simulink model "IEEE30_case"  (R2024b)
settings: Solver=FixedStepAuto  StartTime=0  StopTime=5  FixedStep=1e-7  RelTol=1e-3
values from neighbouring files (symbols this model uses):
  GFL_DFIG_7_C_bus = 0.08    [IEEE30_case_parameters.m]
  GFL_DFIG_7_D_mutual = 2.500000e+3    (= 2500)    [IEEE30_case_parameters.m]
  GFL_DFIG_7_f0 = 60    [IEEE30_case_parameters.m]
  GFL_DFIG_7_gPLLi = 3200    [IEEE30_case_parameters.m]
  GFL_DFIG_7_gPLLp = 650    [IEEE30_case_parameters.m]
  GFL_DFIG_7_H_WT = 0.4    [IEEE30_case_parameters.m]
  GFL_DFIG_7_Hg = 0.8    [IEEE30_case_parameters.m]
  GFL_DFIG_7_Igq_ref = 0    [IEEE30_case_parameters.m]
  GFL_DFIG_7_Ird_ref = 704.45696    [IEEE30_case_parameters.m]
  GFL_DFIG_7_KI_V = -300000    [IEEE30_case_parameters.m]
  GFL_DFIG_7_KP_V = -1000    [IEEE30_case_parameters.m]
  GFL_DFIG_7_Ksh = 1.254300e+4    (= 12543)    [IEEE30_case_parameters.m]
  GFL_DFIG_7_Lg = 0.000483    [IEEE30_case_parameters.m]
  GFL_DFIG_7_Lm_pu = 4    [IEEE30_case_parameters.m]
  GFL_DFIG_7_N = 100    [IEEE30_case_parameters.m]
  GFL_DFIG_7_p = 2    [IEEE30_case_parameters.m]
  GFL_DFIG_7_Pitch = 0    [IEEE30_case_parameters.m]
  GFL_DFIG_7_R = 44    [IEEE30_case_parameters.m]
  GFL_DFIG_7_Rg = 2.000000e-5    (= 2e-05)    [IEEE30_case_parameters.m]
  GFL_DFIG_7_rho = 1.225    [IEEE30_case_parameters.m]
  GFL_DFIG_7_rPLLi = 4500    [IEEE30_case_parameters.m]
  GFL_DFIG_7_rPLLp = 620    [IEEE30_case_parameters.m]
  GFL_DFIG_7_Rs_pu = 0.011    [IEEE30_case_parameters.m]
  GFL_DFIG_7_Sbase = 2.000000e+6    (= 2000000)    [IEEE30_case_parameters.m]
  GFL_DFIG_7_ugq_ref = 0    [IEEE30_case_parameters.m]
  GFL_DFIG_7_usd_ref = 0    [IEEE30_case_parameters.m]
  GFL_DFIG_7_Vbase = 690    [IEEE30_case_parameters.m]
  GFL_DFIG_7_Vdc_ref = 1200    [IEEE30_case_parameters.m]
  GFL_DFIG_7_wind = 12    [IEEE30_case_parameters.m]
  GFL_DFIG_7_wm_ref = 518.184209    [IEEE30_case_parameters.m]
  SG_D_13_D = 0.01056    [IEEE30_case_parameters.m]
  SG_D_13_EnableSaturation = 0    [IEEE30_case_parameters.m]
  SG_D_13_f0 = 60    [IEEE30_case_parameters.m]
  SG_D_13_H = 7.5    [IEEE30_case_parameters.m]
  SG_D_13_K_A = 20    [IEEE30_case_parameters.m]
  SG_D_13_K_E = 1.000000e+1    (= 10)    [IEEE30_case_parameters.m]
  SG_D_13_K_F = 2.363    [IEEE30_case_parameters.m]
  SG_D_13_K_s = 0.5    [IEEE30_case_parameters.m]
  SG_D_13_R_a = 0.001088    [IEEE30_case_parameters.m]
  SG_D_13_S_A = 1    [IEEE30_case_parameters.m]
  SG_D_13_S_B = 0.103    [IEEE30_case_parameters.m]
  SG_D_13_S_N = 10.659857    [IEEE30_case_parameters.m]
  SG_D_13_SpeedPara = 200    [IEEE30_case_parameters.m]
  SG_D_13_T_0 = 0.370163    [IEEE30_case_parameters.m]
  SG_D_13_T_1 = 0.3    [IEEE30_case_parameters.m]
  SG_D_13_T_2 = 0.05    [IEEE30_case_parameters.m]
  SG_D_13_T_3 = 0.02    [IEEE30_case_parameters.m]
  SG_D_13_T_4 = 0.005    [IEEE30_case_parameters.m]
  SG_D_13_T_A = 0.02    [IEEE30_case_parameters.m]
  SG_D_13_T_dd = 8.000000e+0    (= 8)    [IEEE30_case_parameters.m]
  SG_D_13_T_ddd = 0.04    [IEEE30_case_parameters.m]
  SG_D_13_T_E = 0.314    [IEEE30_case_parameters.m]
  SG_D_13_T_F = 0.35    [IEEE30_case_parameters.m]
  SG_D_13_T_qd = 0.8    [IEEE30_case_parameters.m]
  SG_D_13_T_qdd = 0.02    [IEEE30_case_parameters.m]
  SG_D_13_T_speed = 0.1    [IEEE30_case_parameters.m]
  SG_D_13_T_w = 0.5    [IEEE30_case_parameters.m]
  SG_D_13_V_ref = 1.696619    [IEEE30_case_parameters.m]
  SG_D_13_w_ref = 376.991118    [IEEE30_case_parameters.m]
  SG_D_13_x_d = 1.9    [IEEE30_case_parameters.m]
  SG_D_13_x_dd = 0.302    [IEEE30_case_parameters.m]
  SG_D_13_x_ddd = 0.204    [IEEE30_case_parameters.m]
  SG_D_13_x_l = 0.05    [IEEE30_case_parameters.m]
  SG_D_13_x_q = 1.3    [IEEE30_case_parameters.m]
  SG_D_13_x_qd = 0.5    [IEEE30_case_parameters.m]
  SG_D_13_x_qdd = 0.3    [IEEE30_case_parameters.m]
  SG_D_1_D = 0.01056    [IEEE30_case_parameters.m]
  SG_D_1_EnableSaturation = 0    [IEEE30_case_parameters.m]
  SG_D_1_f0 = 60    [IEEE30_case_parameters.m]
  SG_D_1_H = 7.5    [IEEE30_case_parameters.m]
  SG_D_1_K_A = 20    [IEEE30_case_parameters.m]
  SG_D_1_K_E = 1.000000e+1    (= 10)    [IEEE30_case_parameters.m]
  SG_D_1_K_F = 2.363    [IEEE30_case_parameters.m]
  SG_D_1_K_s = 0.5    [IEEE30_case_parameters.m]
  SG_D_1_R_a = 0.001088    [IEEE30_case_parameters.m]
  SG_D_1_S_A = 1    [IEEE30_case_parameters.m]
  SG_D_1_S_B = 0.103    [IEEE30_case_parameters.m]
  SG_D_1_S_N = 10.659857    [IEEE30_case_parameters.m]
  SG_D_1_SpeedPara = 200    [IEEE30_case_parameters.m]
  SG_D_1_T_0 = 0.259812    [IEEE30_case_parameters.m]
  SG_D_1_T_1 = 0.3    [IEEE30_case_parameters.m]
  SG_D_1_T_2 = 0.05    [IEEE30_case_parameters.m]
  SG_D_1_T_3 = 0.02    [IEEE30_case_parameters.m]
  SG_D_1_T_4 = 0.005    [IEEE30_case_parameters.m]
  SG_D_1_T_A = 0.02    [IEEE30_case_parameters.m]
  SG_D_1_T_dd = 8.000000e+0    (= 8)    [IEEE30_case_parameters.m]
  SG_D_1_T_ddd = 0.04    [IEEE30_case_parameters.m]
  SG_D_1_T_E = 0.314    [IEEE30_case_parameters.m]
  SG_D_1_T_F = 0.35    [IEEE30_case_parameters.m]
  SG_D_1_T_qd = 0.8    [IEEE30_case_parameters.m]
  SG_D_1_T_qdd = 0.02    [IEEE30_case_parameters.m]
  SG_D_1_T_speed = 0.1    [IEEE30_case_parameters.m]
  SG_D_1_T_w = 0.5    [IEEE30_case_parameters.m]
  SG_D_1_V_ref = 1.544107    [IEEE30_case_parameters.m]
  SG_D_1_w_ref = 376.991118    [IEEE30_case_parameters.m]
  SG_D_1_x_d = 1.9    [IEEE30_case_parameters.m]
  SG_D_1_x_dd = 0.302    [IEEE30_case_parameters.m]
  SG_D_1_x_ddd = 0.204    [IEEE30_case_parameters.m]
  SG_D_1_x_l = 0.05    [IEEE30_case_parameters.m]
  SG_D_1_x_q = 1.3    [IEEE30_case_parameters.m]
  SG_D_1_x_qd = 0.5    [IEEE30_case_parameters.m]
  SG_D_1_x_qdd = 0.3    [IEEE30_case_parameters.m]
  SG_D_22_D = 0.01056    [IEEE30_case_parameters.m]
  SG_D_22_EnableSaturation = 0    [IEEE30_case_parameters.m]
  SG_D_22_f0 = 60    [IEEE30_case_parameters.m]
  SG_D_22_H = 7.5    [IEEE30_case_parameters.m]
  SG_D_22_K_A = 20    [IEEE30_case_parameters.m]
  SG_D_22_K_E = 1.000000e+1    (= 10)    [IEEE30_case_parameters.m]
  SG_D_22_K_F = 2.363    [IEEE30_case_parameters.m]
  SG_D_22_K_s = 0.5    [IEEE30_case_parameters.m]
  SG_D_22_R_a = 0.001088    [IEEE30_case_parameters.m]
  SG_D_22_S_A = 1    [IEEE30_case_parameters.m]
  SG_D_22_S_B = 0.103    [IEEE30_case_parameters.m]
  SG_D_22_S_N = 10.659857    [IEEE30_case_parameters.m]
  SG_D_22_SpeedPara = 200    [IEEE30_case_parameters.m]
  SG_D_22_T_0 = 0.216121    [IEEE30_case_parameters.m]
  SG_D_22_T_1 = 0.3    [IEEE30_case_parameters.m]
  SG_D_22_T_2 = 0.05    [IEEE30_case_parameters.m]
  SG_D_22_T_3 = 0.02    [IEEE30_case_parameters.m]
  SG_D_22_T_4 = 0.005    [IEEE30_case_parameters.m]
  ... (+126 more)
(part 9 of 27)

== system IEEE30_case/AC_1/d_iq_load_4_block ==
  note: d_iq_load_4 in IEEE30_case
      | $147.957809890804\,\mathrm{vq}_{\mathrm{bus},4}-1790.70781254618\,\mathrm{iq}_{\mathrm{load},4}-376.991118430775\,\mathrm{id}_{\mathrm{load},4}$
      | Automatically generated on 2025-11-01 18:40:20 .
  State_id_load_4_5343f : Inport
  State_iq_load_4_cbd44 : Inport  Port=2
  State_vq_bus_4_cd35f : Inport  Port=3
  Add_1e4f1 : Sum
  Constant_-376.991118430775_9cf5e : Constant  Value=-376.991118430775
  Constant_147.957809890804_5bb2c : Constant  Value=147.957809890804
  Constant_1790.70781254618_4e840 : Constant  Value=1790.70781254618
  Product_380a7 : Product
  Product_6bb72 : Product
  Product_f426a : Product
  Subtract_c5176 : Sum  Inputs=+-
  Blockout_d_iq_load_4_2d77b : Outport
  wires:
  Constant_-376.991118430775_9cf5e/1 -> Product_f426a/1
  Constant_1790.70781254618_4e840/1 -> Product_6bb72/1
  Product_6bb72/1 -> Subtract_c5176/2
  State_id_load_4_5343f/1 -> Product_f426a/2
  State_iq_load_4_cbd44/1 -> Product_6bb72/2
  Product_f426a/1 -> Subtract_c5176/1
  Constant_147.957809890804_5bb2c/1 -> Product_380a7/1
  State_vq_bus_4_cd35f/1 -> Product_380a7/2
  Subtract_c5176/1 -> Add_1e4f1/1
  Product_380a7/1 -> Add_1e4f1/2
  Add_1e4f1/1 -> Blockout_d_iq_load_4_2d77b/1

== system IEEE30_case/AC_1/d_iq_load_7_block ==
  note: d_iq_load_7 in IEEE30_case
      | $441.543140918512\,\mathrm{vq}_{\mathrm{bus},7}-1134.43198940637\,\mathrm{iq}_{\mathrm{load},7}-376.991118430775\,\mathrm{id}_{\mathrm{load},7}$
      | Automatically generated on 2025-11-01 18:40:22 .
  State_id_load_7_bd96d : Inport
  State_iq_load_7_42ee7 : Inport  Port=2
  State_vq_bus_7_bc847 : Inport  Port=3
  Add_c31b1 : Sum
  Constant_-376.991118430775_3d6e2 : Constant  Value=-376.991118430775
  Constant_1134.43198940637_2d126 : Constant  Value=1134.43198940637
  Constant_441.543140918512_88dfd : Constant  Value=441.543140918512
  Product_1255a : Product
  Product_502dd : Product
  Product_66157 : Product
  Subtract_541c0 : Sum  Inputs=+-
  Blockout_d_iq_load_7_f7ad2 : Outport
  wires:
  State_id_load_7_bd96d/1 -> Product_66157/2
  Constant_-376.991118430775_3d6e2/1 -> Product_66157/1
  Constant_1134.43198940637_2d126/1 -> Product_1255a/1
  Product_1255a/1 -> Subtract_541c0/2
  State_iq_load_7_42ee7/1 -> Product_1255a/2
  Product_66157/1 -> Subtract_541c0/1
  Constant_441.543140918512_88dfd/1 -> Product_502dd/1
  State_vq_bus_7_bc847/1 -> Product_502dd/2
  Subtract_541c0/1 -> Add_c31b1/1
  Product_502dd/1 -> Add_c31b1/2
  Add_c31b1/1 -> Blockout_d_iq_load_7_f7ad2/1

== system IEEE30_case/AC_1/d_iq_load_8_block ==
  note: d_iq_load_8 in IEEE30_case
      | $245.118316875829\,\mathrm{vq}_{\mathrm{bus},8}-376.991118430775\,\mathrm{iq}_{\mathrm{load},8}-376.991118430775\,\mathrm{id}_{\mathrm{load},8}$
      | Automatically generated on 2025-11-01 18:40:24 .
  State_id_load_8_a69c1 : Inport
  State_iq_load_8_f08e9 : Inport  Port=2
  State_vq_bus_8_10b00 : Inport  Port=3
  Add_9d265 : Sum
  Constant_-376.991118430775_c6f2d : Constant  Value=-376.991118430775
  Constant_245.118316875829_8cff8 : Constant  Value=245.118316875829
  Constant_376.991118430775_a3b3a : Constant  Value=376.991118430775
  Product_2c64e : Product
  Product_4f060 : Product
  Product_c2130 : Product
  Subtract_7f566 : Sum  Inputs=+-
  Blockout_d_iq_load_8_09960 : Outport
  wires:
  Constant_-376.991118430775_c6f2d/1 -> Product_c2130/1
  State_id_load_8_a69c1/1 -> Product_c2130/2
  Constant_376.991118430775_a3b3a/1 -> Product_2c64e/1
  Product_2c64e/1 -> Subtract_7f566/2
  State_iq_load_8_f08e9/1 -> Product_2c64e/2
  Product_c2130/1 -> Subtract_7f566/1
  Constant_245.118316875829_8cff8/1 -> Product_4f060/1
  State_vq_bus_8_10b00/1 -> Product_4f060/2
  Subtract_7f566/1 -> Add_9d265/1
  Product_4f060/1 -> Add_9d265/2
  Add_9d265/1 -> Blockout_d_iq_load_8_09960/1

== system IEEE30_case/AC_1/d_vd_bus_10_block ==
  note: d_vd_bus_10 in IEEE30_case
      | $37699111.8430775\,\mathrm{id}_{\mathrm{bus},10}+376.991118430775\,\mathrm{vq}_{\mathrm{bus},10}$
      | Automatically generated on 2025-11-01 18:39:38 .
  Alge_id_bus_10_55824 : Inport
  State_vq_bus_10_0727d : Inport  Port=2
  Add_d2c16 : Sum
  Constant_376.991118430775_e5185 : Constant  Value=376.991118430775
  Constant_37699111.8430775_935e5 : Constant  Value=37699111.8430775
  Product_272a3 : Product
  Product_d7e31 : Product
  Blockout_d_vd_bus_10_946a6 : Outport
  wires:
  Constant_37699111.8430775_935e5/1 -> Product_272a3/1
  Alge_id_bus_10_55824/1 -> Product_272a3/2
  Product_d7e31/1 -> Add_d2c16/2
  State_vq_bus_10_0727d/1 -> Product_d7e31/2
  Constant_376.991118430775_e5185/1 -> Product_d7e31/1
  Product_272a3/1 -> Add_d2c16/1
  Add_d2c16/1 -> Blockout_d_vd_bus_10_946a6/1

== system IEEE30_case/AC_1/d_vd_bus_11_block ==
  note: d_vd_bus_11 in IEEE30_case
      | $37699111.8430775\,\mathrm{id}_{\mathrm{bus},11}+376.991118430775\,\mathrm{vq}_{\mathrm{bus},11}$
      | Automatically generated on 2025-11-01 18:39:40 .
  Alge_id_bus_11_02d21 : Inport
  State_vq_bus_11_56182 : Inport  Port=2
  Add_b6a8b : Sum
  Constant_376.991118430775_a35fb : Constant  Value=376.991118430775
  Constant_37699111.8430775_0f988 : Constant  Value=37699111.8430775
  Product_6dfd0 : Product
  Product_d5ffb : Product
  Blockout_d_vd_bus_11_c002c : Outport
  wires:
  Constant_37699111.8430775_0f988/1 -> Product_d5ffb/1
  Product_6dfd0/1 -> Add_b6a8b/2
  Constant_376.991118430775_a35fb/1 -> Product_6dfd0/1
  Alge_id_bus_11_02d21/1 -> Product_d5ffb/2
  State_vq_bus_11_56182/1 -> Product_6dfd0/2
  Product_d5ffb/1 -> Add_b6a8b/1
  Add_b6a8b/1 -> Blockout_d_vd_bus_11_c002c/1

== system IEEE30_case/AC_1/d_vd_bus_12_block ==
  note: d_vd_bus_12 in IEEE30_case
      | $37699111.8430775\,\mathrm{id}_{\mathrm{bus},12}+376.991118430775\,\mathrm{vq}_{\mathrm{bus},12}$
      | Automatically generated on 2025-11-01 18:39:42 .
  Alge_id_bus_12_e0ed8 : Inport
  State_vq_bus_12_edbb2 : Inport  Port=2
  Add_a50b9 : Sum
  Constant_376.991118430775_69f03 : Constant  Value=376.991118430775
  Constant_37699111.8430775_b1ec6 : Constant  Value=37699111.8430775
  Product_5a627 : Product
  Product_de458 : Product
  Blockout_d_vd_bus_12_8eaf3 : Outport
  wires:
  Alge_id_bus_12_e0ed8/1 -> Product_de458/2
  Constant_37699111.8430775_b1ec6/1 -> Product_de458/1
  Constant_376.991118430775_69f03/1 -> Product_5a627/1
  State_vq_bus_12_edbb2/1 -> Product_5a627/2
  Product_de458/1 -> Add_a50b9/1
  Product_5a627/1 -> Add_a50b9/2
  Add_a50b9/1 -> Blockout_d_vd_bus_12_8eaf3/1

== system IEEE30_case/AC_1/d_vd_bus_13_block ==
  note: d_vd_bus_13 in IEEE30_case
      | $37699111.8430775\,\mathrm{id}_{\mathrm{bus},13}+376.991118430775\,\mathrm{vq}_{\mathrm{bus},13}$
      | Automatically generated on 2025-11-01 18:39:43 .
  Alge_id_bus_13_da285 : Inport
  State_vq_bus_13_d83fb : Inport  Port=2
  Add_3b63a : Sum
  Constant_376.991118430775_06774 : Constant  Value=376.991118430775
  Constant_37699111.8430775_bfe4b : Constant  Value=37699111.8430775
  Product_b6505 : Product
  Product_d61ea : Product
  Blockout_d_vd_bus_13_93e1c : Outport
  wires:
  Add_3b63a/1 -> Blockout_d_vd_bus_13_93e1c/1
  Constant_37699111.8430775_bfe4b/1 -> Product_d61ea/1
  Alge_id_bus_13_da285/1 -> Product_d61ea/2
  Product_b6505/1 -> Add_3b63a/2
  Constant_376.991118430775_06774/1 -> Product_b6505/1
  Product_d61ea/1 -> Add_3b63a/1
  State_vq_bus_13_d83fb/1 -> Product_b6505/2

== system IEEE30_case/AC_1/d_vd_bus_14_block ==
  note: d_vd_bus_14 in IEEE30_case
      | $37699111.8430775\,\mathrm{id}_{\mathrm{bus},14}+376.991118430775\,\mathrm{vq}_{\mathrm{bus},14}$
      | Automatically generated on 2025-11-01 18:39:45 .
  Alge_id_bus_14_c396c : Inport
  State_vq_bus_14_a6726 : Inport  Port=2
  Add_b40e3 : Sum
  Constant_376.991118430775_19aab : Constant  Value=376.991118430775
  Constant_37699111.8430775_49935 : Constant  Value=37699111.8430775
  Product_1457a : Product
  Product_b17bc : Product
  Blockout_d_vd_bus_14_5026c : Outport
  wires:
  Constant_37699111.8430775_49935/1 -> Product_1457a/1
  Alge_id_bus_14_c396c/1 -> Product_1457a/2
  Product_b17bc/1 -> Add_b40e3/2
  Constant_376.991118430775_19aab/1 -> Product_b17bc/1
  State_vq_bus_14_a6726/1 -> Product_b17bc/2
  Product_1457a/1 -> Add_b40e3/1
  Add_b40e3/1 -> Blockout_d_vd_bus_14_5026c/1

== system IEEE30_case/AC_1/d_vd_bus_15_block ==
  note: d_vd_bus_15 in IEEE30_case
      | $37699111.8430775\,\mathrm{id}_{\mathrm{bus},15}+376.991118430775\,\mathrm{vq}_{\mathrm{bus},15}$
      | Automatically generated on 2025-11-01 18:39:47 .
  Alge_id_bus_15_5fc28 : Inport
  State_vq_bus_15_cc2ed : Inport  Port=2
  Add_fcc08 : Sum
  Constant_376.991118430775_b3a57 : Constant  Value=376.991118430775
  Constant_37699111.8430775_9ca24 : Constant  Value=37699111.8430775
  Product_37295 : Product
  Product_b793c : Product
  Blockout_d_vd_bus_15_eaf4b : Outport
  wires:
  Add_fcc08/1 -> Blockout_d_vd_bus_15_eaf4b/1
  Constant_37699111.8430775_9ca24/1 -> Product_37295/1
  Alge_id_bus_15_5fc28/1 -> Product_37295/2
  Product_b793c/1 -> Add_fcc08/2
  Constant_376.991118430775_b3a57/1 -> Product_b793c/1
  Product_37295/1 -> Add_fcc08/1
  State_vq_bus_15_cc2ed/1 -> Product_b793c/2

== system IEEE30_case/AC_1/d_vd_bus_16_block ==
  note: d_vd_bus_16 in IEEE30_case
      | $37699111.8430775\,\mathrm{id}_{\mathrm{bus},16}+376.991118430775\,\mathrm{vq}_{\mathrm{bus},16}$
      | Automatically generated on 2025-11-01 18:39:48 .
  Alge_id_bus_16_f0bf0 : Inport
  State_vq_bus_16_133e3 : Inport  Port=2
  Add_6bfbe : Sum
  Constant_376.991118430775_30b31 : Constant  Value=376.991118430775
  Constant_37699111.8430775_fcaaf : Constant  Value=37699111.8430775
  Product_17a02 : Product
  Product_d3068 : Product
  Blockout_d_vd_bus_16_30db1 : Outport
  wires:
  Constant_37699111.8430775_fcaaf/1 -> Product_d3068/1
  Constant_376.991118430775_30b31/1 -> Product_17a02/1
  Alge_id_bus_16_f0bf0/1 -> Product_d3068/2
  Product_17a02/1 -> Add_6bfbe/2
  State_vq_bus_16_133e3/1 -> Product_17a02/2
  Product_d3068/1 -> Add_6bfbe/1
  Add_6bfbe/1 -> Blockout_d_vd_bus_16_30db1/1

== system IEEE30_case/AC_1/d_vd_bus_17_block ==
  note: d_vd_bus_17 in IEEE30_case
      | $37699111.8430775\,\mathrm{id}_{\mathrm{bus},17}+376.991118430775\,\mathrm{vq}_{\mathrm{bus},17}$
      | Automatically generated on 2025-11-01 18:39:50 .
  Alge_id_bus_17_92d80 : Inport
  State_vq_bus_17_c3ce6 : Inport  Port=2
  Add_417f6 : Sum
  Constant_376.991118430775_6f0ab : Constant  Value=376.991118430775
  Constant_37699111.8430775_0b194 : Constant  Value=37699111.8430775
  Product_756d1 : Product
  Product_c8b73 : Product
  Blockout_d_vd_bus_17_9b1fc : Outport
  wires:
  Constant_37699111.8430775_0b194/1 -> Product_756d1/1
  Product_c8b73/1 -> Add_417f6/2
  Constant_376.991118430775_6f0ab/1 -> Product_c8b73/1
  Alge_id_bus_17_92d80/1 -> Product_756d1/2
  State_vq_bus_17_c3ce6/1 -> Product_c8b73/2
  Product_756d1/1 -> Add_417f6/1
  Add_417f6/1 -> Blockout_d_vd_bus_17_9b1fc/1

== system IEEE30_case/AC_1/d_vd_bus_18_block ==
  note: d_vd_bus_18 in IEEE30_case
      | $37699111.8430775\,\mathrm{id}_{\mathrm{bus},18}+376.991118430775\,\mathrm{vq}_{\mathrm{bus},18}$
      | Automatically generated on 2025-11-01 18:39:52 .
  Alge_id_bus_18_7cead : Inport
  State_vq_bus_18_b1f41 : Inport  Port=2
  Add_c3a10 : Sum
  Constant_376.991118430775_7c003 : Constant  Value=376.991118430775
  Constant_37699111.8430775_e7a38 : Constant  Value=37699111.8430775
  Product_10ccb : Product
  Product_7e1ce : Product
  Blockout_d_vd_bus_18_c0af9 : Outport
  wires:
  Constant_37699111.8430775_e7a38/1 -> Product_10ccb/1
  Alge_id_bus_18_7cead/1 -> Product_10ccb/2
  Product_7e1ce/1 -> Add_c3a10/2
  Constant_376.991118430775_7c003/1 -> Product_7e1ce/1
  State_vq_bus_18_b1f41/1 -> Product_7e1ce/2
  Product_10ccb/1 -> Add_c3a10/1
  Add_c3a10/1 -> Blockout_d_vd_bus_18_c0af9/1

== system IEEE30_case/AC_1/d_vd_bus_19_block ==
  note: d_vd_bus_19 in IEEE30_case
      | $37699111.8430775\,\mathrm{id}_{\mathrm{bus},19}+376.991118430775\,\mathrm{vq}_{\mathrm{bus},19}$
      | Automatically generated on 2025-11-01 18:39:53 .
  Alge_id_bus_19_2b5fc : Inport
  State_vq_bus_19_a5c18 : Inport  Port=2
  Add_525dd : Sum
  Constant_376.991118430775_b67bc : Constant  Value=376.991118430775
  Constant_37699111.8430775_43d26 : Constant  Value=37699111.8430775
  Product_2e51c : Product
  Product_6f9d5 : Product
  Blockout_d_vd_bus_19_c546e : Outport
  wires:
  Add_525dd/1 -> Blockout_d_vd_bus_19_c546e/1
  Constant_37699111.8430775_43d26/1 -> Product_2e51c/1
  Alge_id_bus_19_2b5fc/1 -> Product_2e51c/2
  Product_6f9d5/1 -> Add_525dd/2
  Constant_376.991118430775_b67bc/1 -> Product_6f9d5/1
  Product_2e51c/1 -> Add_525dd/1
  State_vq_bus_19_a5c18/1 -> Product_6f9d5/2

== system IEEE30_case/AC_1/d_vd_bus_1_block ==
  note: d_vd_bus_1 in IEEE30_case
      | $15079.644737231\,\mathrm{id}_{\mathrm{bus},1}+376.991118430775\,\mathrm{vq}_{\mathrm{bus},1}$
      | Automatically generated on 2025-11-01 18:39:23 .
  Alge_id_bus_1_1678c : Inport
  State_vq_bus_1_acb41 : Inport  Port=2
  Add_8b1d4 : Sum
  Constant_15079.644737231_7635a : Constant  Value=15079.644737231
  Constant_376.991118430775_3da79 : Constant  Value=376.991118430775
  Product_05e64 : Product
  Product_47af2 : Product
  Blockout_d_vd_bus_1_200d9 : Outport
  wires:
  Constant_15079.644737231_7635a/1 -> Product_47af2/1
  Product_05e64/1 -> Add_8b1d4/2
  Constant_376.991118430775_3da79/1 -> Product_05e64/1
  Alge_id_bus_1_1678c/1 -> Product_47af2/2
  State_vq_bus_1_acb41/1 -> Product_05e64/2
  Product_47af2/1 -> Add_8b1d4/1
  Add_8b1d4/1 -> Blockout_d_vd_bus_1_200d9/1

== system IEEE30_case/AC_1/d_vd_bus_20_block ==
  note: d_vd_bus_20 in IEEE30_case
      | $37699111.8430775\,\mathrm{id}_{\mathrm{bus},20}+376.991118430775\,\mathrm{vq}_{\mathrm{bus},20}$
      | Automatically generated on 2025-11-01 18:39:55 .
  Alge_id_bus_20_5519e : Inport
  State_vq_bus_20_f55e8 : Inport  Port=2
  Add_b62a7 : Sum
  Constant_376.991118430775_89860 : Constant  Value=376.991118430775
  Constant_37699111.8430775_fce1e : Constant  Value=37699111.8430775
  Product_1ab34 : Product
  Product_fa8d5 : Product
  Blockout_d_vd_bus_20_bf639 : Outport
  wires:
  Add_b62a7/1 -> Blockout_d_vd_bus_20_bf639/1
  Constant_37699111.8430775_fce1e/1 -> Product_1ab34/1
  Alge_id_bus_20_5519e/1 -> Product_1ab34/2
  Constant_376.991118430775_89860/1 -> Product_fa8d5/1
  Product_1ab34/1 -> Add_b62a7/1
  State_vq_bus_20_f55e8/1 -> Product_fa8d5/2
  Product_fa8d5/1 -> Add_b62a7/2

== system IEEE30_case/AC_1/d_vd_bus_21_block ==
  note: d_vd_bus_21 in IEEE30_case
      | $37699111.8430775\,\mathrm{id}_{\mathrm{bus},21}+376.991118430775\,\mathrm{vq}_{\mathrm{bus},21}$
      | Automatically generated on 2025-11-01 18:39:57 .
  Alge_id_bus_21_08784 : Inport
  State_vq_bus_21_fbe4c : Inport  Port=2
  Add_8df8c : Sum
  Constant_376.991118430775_7fe5b : Constant  Value=376.991118430775
  Constant_37699111.8430775_0cb98 : Constant  Value=37699111.8430775
  Product_7cee3 : Product
  Product_d338b : Product
  Blockout_d_vd_bus_21_3eacf : Outport
  wires:
  Constant_37699111.8430775_0cb98/1 -> Product_d338b/1
  Alge_id_bus_21_08784/1 -> Product_d338b/2
  Product_7cee3/1 -> Add_8df8c/2
  State_vq_bus_21_fbe4c/1 -> Product_7cee3/2
  Constant_376.991118430775_7fe5b/1 -> Product_7cee3/1
  Product_d338b/1 -> Add_8df8c/1
  Add_8df8c/1 -> Blockout_d_vd_bus_21_3eacf/1

== system IEEE30_case/AC_1/d_vd_bus_22_block ==
  note: d_vd_bus_22 in IEEE30_case
      | $37699111.8430775\,\mathrm{id}_{\mathrm{bus},22}+376.991118430775\,\mathrm{vq}_{\mathrm{bus},22}$
      | Automatically generated on 2025-11-01 18:39:59 .
  Alge_id_bus_22_6e14d : Inport
  State_vq_bus_22_93f74 : Inport  Port=2
  Add_b7e32 : Sum
  Constant_376.991118430775_ac6fe : Constant  Value=376.991118430775
  Constant_37699111.8430775_63bb5 : Constant  Value=37699111.8430775
  Product_34761 : Product
  Product_d02d3 : Product
  Blockout_d_vd_bus_22_f19b2 : Outport
  wires:
  Add_b7e32/1 -> Blockout_d_vd_bus_22_f19b2/1
  Constant_37699111.8430775_63bb5/1 -> Product_34761/1
  Alge_id_bus_22_6e14d/1 -> Product_34761/2
  Product_d02d3/1 -> Add_b7e32/2
  Constant_376.991118430775_ac6fe/1 -> Product_d02d3/1
  State_vq_bus_22_93f74/1 -> Product_d02d3/2
  Product_34761/1 -> Add_b7e32/1

== system IEEE30_case/AC_1/d_vd_bus_23_block ==
  note: d_vd_bus_23 in IEEE30_case
      | $37699111.8430775\,\mathrm{id}_{\mathrm{bus},23}+376.991118430775\,\mathrm{vq}_{\mathrm{bus},23}$
      | Automatically generated on 2025-11-01 18:40:00 .
  Alge_id_bus_23_3d01a : Inport
  State_vq_bus_23_506e6 : Inport  Port=2
  Add_c66b6 : Sum
  Constant_376.991118430775_5be61 : Constant  Value=376.991118430775
  Constant_37699111.8430775_11e28 : Constant  Value=37699111.8430775
  Product_8f7d7 : Product
  Product_c4ca6 : Product
  Blockout_d_vd_bus_23_d2881 : Outport
  wires:
  Add_c66b6/1 -> Blockout_d_vd_bus_23_d2881/1
  Constant_37699111.8430775_11e28/1 -> Product_c4ca6/1
  Alge_id_bus_23_3d01a/1 -> Product_c4ca6/2
  Product_8f7d7/1 -> Add_c66b6/2
  Constant_376.991118430775_5be61/1 -> Product_8f7d7/1
  Product_c4ca6/1 -> Add_c66b6/1
  State_vq_bus_23_506e6/1 -> Product_8f7d7/2

== system IEEE30_case/AC_1/d_vd_bus_24_block ==
  note: d_vd_bus_24 in IEEE30_case
      | $942477.796076938\,\mathrm{id}_{\mathrm{bus},24}+376.991118430775\,\mathrm{vq}_{\mathrm{bus},24}$
      | Automatically generated on 2025-11-01 18:40:02 .
  Alge_id_bus_24_d1ab9 : Inport
  State_vq_bus_24_3465a : Inport  Port=2
  Add_d2fef : Sum
  Constant_376.991118430775_cdf8d : Constant  Value=376.991118430775
  Constant_942477.796076938_11872 : Constant  Value=942477.796076938
  Product_12591 : Product
  Product_69bed : Product
  Blockout_d_vd_bus_24_09370 : Outport
  wires:
  Constant_942477.796076938_11872/1 -> Product_69bed/1
  Constant_376.991118430775_cdf8d/1 -> Product_12591/1
  Alge_id_bus_24_d1ab9/1 -> Product_69bed/2
  Product_12591/1 -> Add_d2fef/2
  State_vq_bus_24_3465a/1 -> Product_12591/2
  Product_69bed/1 -> Add_d2fef/1
  Add_d2fef/1 -> Blockout_d_vd_bus_24_09370/1

== system IEEE30_case/AC_1/d_vd_bus_25_block ==
  note: d_vd_bus_25 in IEEE30_case
      | $37699111.8430775\,\mathrm{id}_{\mathrm{bus},25}+376.991118430775\,\mathrm{vq}_{\mathrm{bus},25}$
      | Automatically generated on 2025-11-01 18:40:04 .
  Alge_id_bus_25_c584c : Inport
  State_vq_bus_25_926f5 : Inport  Port=2
  Add_725c4 : Sum
  Constant_376.991118430775_6577a : Constant  Value=376.991118430775
  Constant_37699111.8430775_15ab3 : Constant  Value=37699111.8430775
  Product_6a823 : Product
  Product_dfb4e : Product
  Blockout_d_vd_bus_25_c0f98 : Outport
  wires:
  Constant_37699111.8430775_15ab3/1 -> Product_6a823/1
  Product_dfb4e/1 -> Add_725c4/2
  Constant_376.991118430775_6577a/1 -> Product_dfb4e/1
  Alge_id_bus_25_c584c/1 -> Product_6a823/2
  State_vq_bus_25_926f5/1 -> Product_dfb4e/2
  Product_6a823/1 -> Add_725c4/1
  Add_725c4/1 -> Blockout_d_vd_bus_25_c0f98/1

== system IEEE30_case/AC_1/d_vd_bus_26_block ==
  note: d_vd_bus_26 in IEEE30_case
      | $37699111.8430775\,\mathrm{id}_{\mathrm{bus},26}+376.991118430775\,\mathrm{vq}_{\mathrm{bus},26}$
      | Automatically generated on 2025-11-01 18:40:06 .
  Alge_id_bus_26_ff4d0 : Inport
  State_vq_bus_26_91c38 : Inport  Port=2
  Add_f7538 : Sum
  Constant_376.991118430775_38254 : Constant  Value=376.991118430775
  Constant_37699111.8430775_3e0e8 : Constant  Value=37699111.8430775
  Product_5992d : Product
  Product_81959 : Product
  Blockout_d_vd_bus_26_d635e : Outport
  wires:
  Constant_37699111.8430775_3e0e8/1 -> Product_81959/1
  Alge_id_bus_26_ff4d0/1 -> Product_81959/2
  Product_5992d/1 -> Add_f7538/2
  Constant_376.991118430775_38254/1 -> Product_5992d/1
  State_vq_bus_26_91c38/1 -> Product_5992d/2
  Product_81959/1 -> Add_f7538/1
  Add_f7538/1 -> Blockout_d_vd_bus_26_d635e/1

== system IEEE30_case/AC_1/d_vd_bus_27_block ==
  note: d_vd_bus_27 in IEEE30_case
      | $37699111.8430775\,\mathrm{id}_{\mathrm{bus},27}+376.991118430775\,\mathrm{vq}_{\mathrm{bus},27}$
      | Automatically generated on 2025-11-01 18:40:07 .
  Alge_id_bus_27_de3da : Inport
  State_vq_bus_27_1ff45 : Inport  Port=2
  Add_83f8f : Sum
  Constant_376.991118430775_97b5c : Constant  Value=376.991118430775
  Constant_37699111.8430775_4fd87 : Constant  Value=37699111.8430775
  Product_0bb53 : Product
  Product_1ae5d : Product
  Blockout_d_vd_bus_27_83d7e : Outport
  wires:
  Add_83f8f/1 -> Blockout_d_vd_bus_27_83d7e/1
  Constant_37699111.8430775_4fd87/1 -> Product_1ae5d/1
  Alge_id_bus_27_de3da/1 -> Product_1ae5d/2
  Product_0bb53/1 -> Add_83f8f/2
  Constant_376.991118430775_97b5c/1 -> Product_0bb53/1
  Product_1ae5d/1 -> Add_83f8f/1
  State_vq_bus_27_1ff45/1 -> Product_0bb53/2

== system IEEE30_case/AC_1/d_vd_bus_28_block ==
  note: d_vd_bus_28 in IEEE30_case
      | $25132.7412287183\,\mathrm{id}_{\mathrm{bus},28}+376.991118430775\,\mathrm{vq}_{\mathrm{bus},28}$
      | Automatically generated on 2025-11-01 18:40:09 .
  Alge_id_bus_28_5e372 : Inport
  State_vq_bus_28_2c3ac : Inport  Port=2
  Add_c3372 : Sum
  Constant_25132.7412287183_580cd : Constant  Value=25132.7412287183
  Constant_376.991118430775_adc65 : Constant  Value=376.991118430775
  Product_a75c1 : Product
  Product_c8b92 : Product
  Blockout_d_vd_bus_28_2c5eb : Outport
  wires:
  Add_c3372/1 -> Blockout_d_vd_bus_28_2c5eb/1
  Constant_25132.7412287183_580cd/1 -> Product_c8b92/1
  Alge_id_bus_28_5e372/1 -> Product_c8b92/2
  Constant_376.991118430775_adc65/1 -> Product_a75c1/1
  Product_c8b92/1 -> Add_c3372/1
  State_vq_bus_28_2c3ac/1 -> Product_a75c1/2
  Product_a75c1/1 -> Add_c3372/2

== system IEEE30_case/AC_1/d_vd_bus_29_block ==
  note: d_vd_bus_29 in IEEE30_case
      | $37699111.8430775\,\mathrm{id}_{\mathrm{bus},29}+376.991118430775\,\mathrm{vq}_{\mathrm{bus},29}$
      | Automatically generated on 2025-11-01 18:40:11 .
  Alge_id_bus_29_eb4d1 : Inport
  State_vq_bus_29_f75e0 : Inport  Port=2
  Add_00bad : Sum
  Constant_376.991118430775_2d4e5 : Constant  Value=376.991118430775
  Constant_37699111.8430775_9f3e6 : Constant  Value=37699111.8430775
  Product_8dd57 : Product
  Product_9890c : Product
  Blockout_d_vd_bus_29_ae863 : Outport
  wires:
  Constant_37699111.8430775_9f3e6/1 -> Product_9890c/1
  State_vq_bus_29_f75e0/1 -> Product_8dd57/2
  Alge_id_bus_29_eb4d1/1 -> Product_9890c/2
  Product_8dd57/1 -> Add_00bad/2
  Constant_376.991118430775_2d4e5/1 -> Product_8dd57/1
  Product_9890c/1 -> Add_00bad/1
  Add_00bad/1 -> Blockout_d_vd_bus_29_ae863/1

== system IEEE30_case/AC_1/d_vd_bus_2_block ==
  note: d_vd_bus_2 in IEEE30_case
      | $8377.58040957278\,\mathrm{id}_{\mathrm{bus},2}+376.991118430775\,\mathrm{vq}_{\mathrm{bus},2}$
      | Automatically generated on 2025-11-01 18:39:25 .
  Alge_id_bus_2_79afc : Inport
  State_vq_bus_2_2b9b5 : Inport  Port=2
  Add_bdae1 : Sum
  Constant_376.991118430775_c005a : Constant  Value=376.991118430775
  Constant_8377.58040957278_a1f87 : Constant  Value=8377.58040957278
  Product_37ffd : Product
  Product_c2bb3 : Product
  Blockout_d_vd_bus_2_2c7da : Outport
  wires:
  Constant_8377.58040957278_a1f87/1 -> Product_37ffd/1
  Alge_id_bus_2_79afc/1 -> Product_37ffd/2
  Product_c2bb3/1 -> Add_bdae1/2
  Constant_376.991118430775_c005a/1 -> Product_c2bb3/1
  State_vq_bus_2_2b9b5/1 -> Product_c2bb3/2
  Product_37ffd/1 -> Add_bdae1/1
  Add_bdae1/1 -> Blockout_d_vd_bus_2_2c7da/1

== system IEEE30_case/AC_1/d_vd_bus_30_block ==
  note: d_vd_bus_30 in IEEE30_case
      | $37699111.8430775\,\mathrm{id}_{\mathrm{bus},30}+376.991118430775\,\mathrm{vq}_{\mathrm{bus},30}$
      | Automatically generated on 2025-11-01 18:40:12 .
  Alge_id_bus_30_9d0e0 : Inport
  State_vq_bus_30_f82c1 : Inport  Port=2
  Add_53dbf : Sum
  Constant_376.991118430775_70e99 : Constant  Value=376.991118430775
  Constant_37699111.8430775_edb54 : Constant  Value=37699111.8430775
  Product_2776c : Product
  Product_34043 : Product
  Blockout_d_vd_bus_30_d4924 : Outport
  wires:
  Constant_37699111.8430775_edb54/1 -> Product_34043/1
  Alge_id_bus_30_9d0e0/1 -> Product_34043/2
  Product_2776c/1 -> Add_53dbf/2
  Constant_376.991118430775_70e99/1 -> Product_2776c/1
  State_vq_bus_30_f82c1/1 -> Product_2776c/2
  Product_34043/1 -> Add_53dbf/1
  Add_53dbf/1 -> Blockout_d_vd_bus_30_d4924/1

== system IEEE30_case/AC_1/d_vd_bus_3_block ==
  note: d_vd_bus_3 in IEEE30_case
      | $37699.1118430775\,\mathrm{id}_{\mathrm{bus},3}+376.991118430775\,\mathrm{vq}_{\mathrm{bus},3}$
      | Automatically generated on 2025-11-01 18:39:26 .
  Alge_id_bus_3_320e9 : Inport
  State_vq_bus_3_0fb23 : Inport  Port=2
  Add_dafc2 : Sum
  Constant_376.991118430775_ce346 : Constant  Value=376.991118430775
  Constant_37699.1118430775_d0604 : Constant  Value=37699.1118430775
  Product_877bd : Product
  Product_a46cb : Product
  Blockout_d_vd_bus_3_b5880 : Outport
  wires:
  Add_dafc2/1 -> Blockout_d_vd_bus_3_b5880/1
  Constant_37699.1118430775_d0604/1 -> Product_a46cb/1
  Alge_id_bus_3_320e9/1 -> Product_a46cb/2
  Product_877bd/1 -> Add_dafc2/2
  Constant_376.991118430775_ce346/1 -> Product_877bd/1
  Product_a46cb/1 -> Add_dafc2/1
  State_vq_bus_3_0fb23/1 -> Product_877bd/2

== system IEEE30_case/AC_1/d_vd_bus_4_block ==
  note: d_vd_bus_4 in IEEE30_case
      | $37699.1118430775\,\mathrm{id}_{\mathrm{bus},4}+376.991118430775\,\mathrm{vq}_{\mathrm{bus},4}$
      | Automatically generated on 2025-11-01 18:39:28 .
  Alge_id_bus_4_472b5 : Inport
  State_vq_bus_4_40a27 : Inport  Port=2
  Add_51f32 : Sum
  Constant_376.991118430775_78fd8 : Constant  Value=376.991118430775
  Constant_37699.1118430775_f9edb : Constant  Value=37699.1118430775
  Product_f1ccc : Product
  Product_f9803 : Product
  Blockout_d_vd_bus_4_76e25 : Outport
  wires:
  Add_51f32/1 -> Blockout_d_vd_bus_4_76e25/1
  Constant_37699.1118430775_f9edb/1 -> Product_f1ccc/1
  Alge_id_bus_4_472b5/1 -> Product_f1ccc/2
  Constant_376.991118430775_78fd8/1 -> Product_f9803/1
  Product_f1ccc/1 -> Add_51f32/1
  State_vq_bus_4_40a27/1 -> Product_f9803/2
  Product_f9803/1 -> Add_51f32/2

== system IEEE30_case/AC_1/d_vd_bus_5_block ==
  note: d_vd_bus_5 in IEEE30_case
      | $22307.1667710518\,\mathrm{id}_{\mathrm{bus},5}+376.991118430775\,\mathrm{vq}_{\mathrm{bus},5}$
      | Automatically generated on 2025-11-01 18:39:30 .
  Alge_id_bus_5_015f0 : Inport
  State_vq_bus_5_87cc9 : Inport  Port=2
  Add_40d2d : Sum
  Constant_22307.1667710518_7177c : Constant  Value=22307.1667710518
  Constant_376.991118430775_9f159 : Constant  Value=376.991118430775
  Product_61b09 : Product
  Product_e8ed8 : Product
  Blockout_d_vd_bus_5_739c0 : Outport
  wires:
  Constant_22307.1667710518_7177c/1 -> Product_61b09/1
  Alge_id_bus_5_015f0/1 -> Product_61b09/2
  Product_e8ed8/1 -> Add_40d2d/2
  State_vq_bus_5_87cc9/1 -> Product_e8ed8/2
  Constant_376.991118430775_9f159/1 -> Product_e8ed8/1
  Product_61b09/1 -> Add_40d2d/1
  Add_40d2d/1 -> Blockout_d_vd_bus_5_739c0/1

== system IEEE30_case/AC_1/d_vd_bus_6_block ==
  note: d_vd_bus_6 in IEEE30_case
      | $18849.5559215388\,\mathrm{id}_{\mathrm{bus},6}+376.991118430775\,\mathrm{vq}_{\mathrm{bus},6}$
      | Automatically generated on 2025-11-01 18:39:31 .
  Alge_id_bus_6_cc19e : Inport
  State_vq_bus_6_b1fab : Inport  Port=2
  Add_f9cb1 : Sum
  Constant_18849.5559215388_2c51a : Constant  Value=18849.5559215388
  Constant_376.991118430775_54f51 : Constant  Value=376.991118430775
  Product_1f5b3 : Product
  Product_26645 : Product
  Blockout_d_vd_bus_6_cb8a2 : Outport
  wires:
  Constant_18849.5559215388_2c51a/1 -> Product_1f5b3/1
  Product_26645/1 -> Add_f9cb1/2
  Constant_376.991118430775_54f51/1 -> Product_26645/1
  Alge_id_bus_6_cc19e/1 -> Product_1f5b3/2
  State_vq_bus_6_b1fab/1 -> Product_26645/2
  Product_1f5b3/1 -> Add_f9cb1/1
  Add_f9cb1/1 -> Blockout_d_vd_bus_6_cb8a2/1

== system IEEE30_case/AC_1/d_vd_bus_7_block ==
  note: d_vd_bus_7 in IEEE30_case
      | $37699.1118430775\,\mathrm{id}_{\mathrm{bus},7}+376.991118430775\,\mathrm{vq}_{\mathrm{bus},7}$
      | Automatically generated on 2025-11-01 18:39:33 .
  Alge_id_bus_7_b77de : Inport
  State_vq_bus_7_f4b0c : Inport  Port=2
  Add_87a0f : Sum
  Constant_376.991118430775_9382e : Constant  Value=376.991118430775
  Constant_37699.1118430775_ff562 : Constant  Value=37699.1118430775
  Product_13721 : Product
  Product_572a8 : Product
  Blockout_d_vd_bus_7_4e9f1 : Outport
  wires:
  Alge_id_bus_7_b77de/1 -> Product_572a8/2
  Constant_37699.1118430775_ff562/1 -> Product_572a8/1
  Product_13721/1 -> Add_87a0f/2
  Constant_376.991118430775_9382e/1 -> Product_13721/1
  State_vq_bus_7_f4b0c/1 -> Product_13721/2
  Product_572a8/1 -> Add_87a0f/1
  Add_87a0f/1 -> Blockout_d_vd_bus_7_4e9f1/1

== system IEEE30_case/AC_1/d_vd_bus_8_block ==
  note: d_vd_bus_8 in IEEE30_case
      | $37699.1118430775\,\mathrm{id}_{\mathrm{bus},8}+376.991118430775\,\mathrm{vq}_{\mathrm{bus},8}$
      | Automatically generated on 2025-11-01 18:39:35 .
  Alge_id_bus_8_ddcea : Inport
  State_vq_bus_8_257eb : Inport  Port=2
  Add_d0ded : Sum
  Constant_376.991118430775_9a873 : Constant  Value=376.991118430775
  Constant_37699.1118430775_ee4b6 : Constant  Value=37699.1118430775
  Product_5e7e4 : Product
  Product_f3d95 : Product
  Blockout_d_vd_bus_8_6724c : Outport
  wires:
  Add_d0ded/1 -> Blockout_d_vd_bus_8_6724c/1
  Constant_37699.1118430775_ee4b6/1 -> Product_5e7e4/1
  Alge_id_bus_8_ddcea/1 -> Product_5e7e4/2
  Constant_376.991118430775_9a873/1 -> Product_f3d95/1
  Product_5e7e4/1 -> Add_d0ded/1
  State_vq_bus_8_257eb/1 -> Product_f3d95/2
  Product_f3d95/1 -> Add_d0ded/2

== system IEEE30_case/AC_1/d_vd_bus_9_block ==
  note: d_vd_bus_9 in IEEE30_case
      | $37699111.8430775\,\mathrm{id}_{\mathrm{bus},9}+376.991118430775\,\mathrm{vq}_{\mathrm{bus},9}$
      | Automatically generated on 2025-11-01 18:39:37 .
  Alge_id_bus_9_9bb77 : Inport
  State_vq_bus_9_a0ae4 : Inport  Port=2
  Add_b9569 : Sum
  Constant_376.991118430775_115d2 : Constant  Value=376.991118430775
  Constant_37699111.8430775_828ab : Constant  Value=37699111.8430775
  Product_12bdd : Product
  Product_56ba0 : Product
  Blockout_d_vd_bus_9_ffce9 : Outport
  wires:
  Add_b9569/1 -> Blockout_d_vd_bus_9_ffce9/1
  Constant_37699111.8430775_828ab/1 -> Product_56ba0/1
  Alge_id_bus_9_9bb77/1 -> Product_56ba0/2
  Product_12bdd/1 -> Add_b9569/2
  Constant_376.991118430775_115d2/1 -> Product_12bdd/1
  Product_56ba0/1 -> Add_b9569/1
  State_vq_bus_9_a0ae4/1 -> Product_12bdd/2

== system IEEE30_case/AC_1/d_vq_bus_10_block ==
  note: d_vq_bus_10 in IEEE30_case
      | $37699111.8430775\,\mathrm{iq}_{\mathrm{bus},10}-376.991118430775\,\mathrm{vd}_{\mathrm{bus},10}$
      | Automatically generated on 2025-11-01 18:39:39 .
  Alge_iq_bus_10_74e9d : Inport
  State_vd_bus_10_649cc : Inport  Port=2
  Constant_376.991118430775_e540e : Constant  Value=376.991118430775
  Constant_37699111.8430775_3e0eb : Constant  Value=37699111.8430775
  Product_09204 : Product
  Product_2f30e : Product
  Subtract_5844f : Sum  Inputs=+-
  Blockout_d_vq_bus_10_d65a2 : Outport
  wires:
  Constant_37699111.8430775_3e0eb/1 -> Product_09204/1
  Alge_iq_bus_10_74e9d/1 -> Product_09204/2
  Constant_376.991118430775_e540e/1 -> Product_2f30e/1
  Product_2f30e/1 -> Subtract_5844f/2
  State_vd_bus_10_649cc/1 -> Product_2f30e/2
  Product_09204/1 -> Subtract_5844f/1
  Subtract_5844f/1 -> Blockout_d_vq_bus_10_d65a2/1

== system IEEE30_case/AC_1/d_vq_bus_11_block ==
  note: d_vq_bus_11 in IEEE30_case
      | $37699111.8430775\,\mathrm{iq}_{\mathrm{bus},11}-376.991118430775\,\mathrm{vd}_{\mathrm{bus},11}$
      | Automatically generated on 2025-11-01 18:39:41 .
  Alge_iq_bus_11_6efd4 : Inport
  State_vd_bus_11_8616a : Inport  Port=2
  Constant_376.991118430775_eece3 : Constant  Value=376.991118430775
  Constant_37699111.8430775_68c47 : Constant  Value=37699111.8430775
  Product_19db2 : Product
  Product_c5ead : Product
  Subtract_78a6e : Sum  Inputs=+-
  Blockout_d_vq_bus_11_520df : Outport
  wires:
  Constant_37699111.8430775_68c47/1 -> Product_19db2/1
  Product_c5ead/1 -> Subtract_78a6e/2
  Constant_376.991118430775_eece3/1 -> Product_c5ead/1
  Alge_iq_bus_11_6efd4/1 -> Product_19db2/2
  State_vd_bus_11_8616a/1 -> Product_c5ead/2
  Product_19db2/1 -> Subtract_78a6e/1
  Subtract_78a6e/1 -> Blockout_d_vq_bus_11_520df/1

== system IEEE30_case/AC_1/d_vq_bus_12_block ==
  note: d_vq_bus_12 in IEEE30_case
      | $37699111.8430775\,\mathrm{iq}_{\mathrm{bus},12}-376.991118430775\,\mathrm{vd}_{\mathrm{bus},12}$
      | Automatically generated on 2025-11-01 18:39:42 .
  Alge_iq_bus_12_c8c41 : Inport
  State_vd_bus_12_a627c : Inport  Port=2
  Constant_376.991118430775_09d4a : Constant  Value=376.991118430775
  Constant_37699111.8430775_7ae84 : Constant  Value=37699111.8430775
  Product_33ce6 : Product
  Product_e3873 : Product
  Subtract_56904 : Sum  Inputs=+-
  Blockout_d_vq_bus_12_c4166 : Outport
  wires:
  Constant_37699111.8430775_7ae84/1 -> Product_33ce6/1
  Alge_iq_bus_12_c8c41/1 -> Product_33ce6/2
  Product_e3873/1 -> Subtract_56904/2
  Constant_376.991118430775_09d4a/1 -> Product_e3873/1
  State_vd_bus_12_a627c/1 -> Product_e3873/2
  Product_33ce6/1 -> Subtract_56904/1
  Subtract_56904/1 -> Blockout_d_vq_bus_12_c4166/1

== system IEEE30_case/AC_1/d_vq_bus_13_block ==
  note: d_vq_bus_13 in IEEE30_case
      | $37699111.8430775\,\mathrm{iq}_{\mathrm{bus},13}-376.991118430775\,\mathrm{vd}_{\mathrm{bus},13}$
      | Automatically generated on 2025-11-01 18:39:44 .
  Alge_iq_bus_13_8e98b : Inport
  State_vd_bus_13_824e9 : Inport  Port=2
  Constant_376.991118430775_f32a4 : Constant  Value=376.991118430775
  Constant_37699111.8430775_b5b5f : Constant  Value=37699111.8430775
  Product_5f19d : Product
  Product_ff46b : Product
  Subtract_ba0b8 : Sum  Inputs=+-
  Blockout_d_vq_bus_13_29628 : Outport
  wires:
  Subtract_ba0b8/1 -> Blockout_d_vq_bus_13_29628/1
  Constant_37699111.8430775_b5b5f/1 -> Product_5f19d/1
  Alge_iq_bus_13_8e98b/1 -> Product_5f19d/2
  Product_ff46b/1 -> Subtract_ba0b8/2
  Constant_376.991118430775_f32a4/1 -> Product_ff46b/1
  Product_5f19d/1 -> Subtract_ba0b8/1
  State_vd_bus_13_824e9/1 -> Product_ff46b/2

== system IEEE30_case/AC_1/d_vq_bus_14_block ==
  note: d_vq_bus_14 in IEEE30_case
      | $37699111.8430775\,\mathrm{iq}_{\mathrm{bus},14}-376.991118430775\,\mathrm{vd}_{\mathrm{bus},14}$
      | Automatically generated on 2025-11-01 18:39:46 .
  Alge_iq_bus_14_fa60c : Inport
  State_vd_bus_14_a89db : Inport  Port=2
  Constant_376.991118430775_c22f7 : Constant  Value=376.991118430775
  Constant_37699111.8430775_85949 : Constant  Value=37699111.8430775
  Product_33f4a : Product
  Product_cc488 : Product
  Subtract_3eb2d : Sum  Inputs=+-
  Blockout_d_vq_bus_14_01909 : Outport
  wires:
  Subtract_3eb2d/1 -> Blockout_d_vq_bus_14_01909/1
  Constant_37699111.8430775_85949/1 -> Product_33f4a/1
  Alge_iq_bus_14_fa60c/1 -> Product_33f4a/2
  Constant_376.991118430775_c22f7/1 -> Product_cc488/1
  Product_33f4a/1 -> Subtract_3eb2d/1
  State_vd_bus_14_a89db/1 -> Product_cc488/2
  Product_cc488/1 -> Subtract_3eb2d/2

== system IEEE30_case/AC_1/d_vq_bus_15_block ==
  note: d_vq_bus_15 in IEEE30_case
      | $37699111.8430775\,\mathrm{iq}_{\mathrm{bus},15}-376.991118430775\,\mathrm{vd}_{\mathrm{bus},15}$
      | Automatically generated on 2025-11-01 18:39:47 .
  Alge_iq_bus_15_10184 : Inport
  State_vd_bus_15_568cb : Inport  Port=2
  Constant_376.991118430775_3694f : Constant  Value=376.991118430775
  Constant_37699111.8430775_ade13 : Constant  Value=37699111.8430775
  Product_5bfa3 : Product
  Product_d4a99 : Product
  Subtract_8eec6 : Sum  Inputs=+-
  Blockout_d_vq_bus_15_2b663 : Outport
  wires:
  Constant_37699111.8430775_ade13/1 -> Product_d4a99/1
  Alge_iq_bus_15_10184/1 -> Product_d4a99/2
  Product_5bfa3/1 -> Subtract_8eec6/2
  State_vd_bus_15_568cb/1 -> Product_5bfa3/2
  Constant_376.991118430775_3694f/1 -> Product_5bfa3/1
  Product_d4a99/1 -> Subtract_8eec6/1
  Subtract_8eec6/1 -> Blockout_d_vq_bus_15_2b663/1

== system IEEE30_case/AC_1/d_vq_bus_16_block ==
  note: d_vq_bus_16 in IEEE30_case
      | $37699111.8430775\,\mathrm{iq}_{\mathrm{bus},16}-376.991118430775\,\mathrm{vd}_{\mathrm{bus},16}$
      | Automatically generated on 2025-11-01 18:39:49 .
  Alge_iq_bus_16_974ba : Inport
  State_vd_bus_16_b3b80 : Inport  Port=2
  Constant_376.991118430775_8d2f1 : Constant  Value=376.991118430775
  Constant_37699111.8430775_8005c : Constant  Value=37699111.8430775
  Product_264a7 : Product
  Product_b44b6 : Product
  Subtract_4c295 : Sum  Inputs=+-
  Blockout_d_vq_bus_16_2931f : Outport
  wires:
  State_vd_bus_16_b3b80/1 -> Product_b44b6/2
  Constant_37699111.8430775_8005c/1 -> Product_264a7/1
  Product_b44b6/1 -> Subtract_4c295/2
  Constant_376.991118430775_8d2f1/1 -> Product_b44b6/1
  Alge_iq_bus_16_974ba/1 -> Product_264a7/2
  Product_264a7/1 -> Subtract_4c295/1
  Subtract_4c295/1 -> Blockout_d_vq_bus_16_2931f/1

== system IEEE30_case/AC_1/d_vq_bus_17_block ==
  note: d_vq_bus_17 in IEEE30_case
      | $37699111.8430775\,\mathrm{iq}_{\mathrm{bus},17}-376.991118430775\,\mathrm{vd}_{\mathrm{bus},17}$
      | Automatically generated on 2025-11-01 18:39:51 .
  Alge_iq_bus_17_e57db : Inport
  State_vd_bus_17_b3717 : Inport  Port=2
  Constant_376.991118430775_023cc : Constant  Value=376.991118430775
  Constant_37699111.8430775_6f865 : Constant  Value=37699111.8430775
  Product_03d3a : Product
  Product_b4696 : Product
  Subtract_fc5ca : Sum  Inputs=+-
  Blockout_d_vq_bus_17_cf2d4 : Outport
  wires:
  Alge_iq_bus_17_e57db/1 -> Product_b4696/2
  Constant_37699111.8430775_6f865/1 -> Product_b4696/1
  Product_03d3a/1 -> Subtract_fc5ca/2
  Constant_376.991118430775_023cc/1 -> Product_03d3a/1
  State_vd_bus_17_b3717/1 -> Product_03d3a/2
  Product_b4696/1 -> Subtract_fc5ca/1
  Subtract_fc5ca/1 -> Blockout_d_vq_bus_17_cf2d4/1

== system IEEE30_case/AC_1/d_vq_bus_18_block ==
  note: d_vq_bus_18 in IEEE30_case
      | $37699111.8430775\,\mathrm{iq}_{\mathrm{bus},18}-376.991118430775\,\mathrm{vd}_{\mathrm{bus},18}$
      | Automatically generated on 2025-11-01 18:39:53 .
  Alge_iq_bus_18_aa760 : Inport
  State_vd_bus_18_3c890 : Inport  Port=2
  Constant_376.991118430775_03ed6 : Constant  Value=376.991118430775
  Constant_37699111.8430775_ff4ab : Constant  Value=37699111.8430775
  Product_17a3c : Product
  Product_7b925 : Product
  Subtract_77419 : Sum  Inputs=+-
  Blockout_d_vq_bus_18_0ee5d : Outport
  wires:
  Subtract_77419/1 -> Blockout_d_vq_bus_18_0ee5d/1
  Constant_37699111.8430775_ff4ab/1 -> Product_7b925/1
  Alge_iq_bus_18_aa760/1 -> Product_7b925/2
  Constant_376.991118430775_03ed6/1 -> Product_17a3c/1
  Product_7b925/1 -> Subtract_77419/1
  State_vd_bus_18_3c890/1 -> Product_17a3c/2
  Product_17a3c/1 -> Subtract_77419/2

== system IEEE30_case/AC_1/d_vq_bus_19_block ==
  note: d_vq_bus_19 in IEEE30_case
      | $37699111.8430775\,\mathrm{iq}_{\mathrm{bus},19}-376.991118430775\,\mathrm{vd}_{\mathrm{bus},19}$
      | Automatically generated on 2025-11-01 18:39:54 .
  Alge_iq_bus_19_ec54b : Inport
  State_vd_bus_19_f463f : Inport  Port=2
  Constant_376.991118430775_faf15 : Constant  Value=376.991118430775
  Constant_37699111.8430775_91faa : Constant  Value=37699111.8430775
  Product_0e411 : Product
  Product_4aa1a : Product
  Subtract_abaaf : Sum  Inputs=+-
  Blockout_d_vq_bus_19_831b3 : Outport
  wires:
  Subtract_abaaf/1 -> Blockout_d_vq_bus_19_831b3/1
  Constant_37699111.8430775_91faa/1 -> Product_4aa1a/1
  Alge_iq_bus_19_ec54b/1 -> Product_4aa1a/2
  Product_0e411/1 -> Subtract_abaaf/2
  Constant_376.991118430775_faf15/1 -> Product_0e411/1
  Product_4aa1a/1 -> Subtract_abaaf/1
  State_vd_bus_19_f463f/1 -> Product_0e411/2

== system IEEE30_case/AC_1/d_vq_bus_1_block ==
  note: d_vq_bus_1 in IEEE30_case
      | $15079.644737231\,\mathrm{iq}_{\mathrm{bus},1}-376.991118430775\,\mathrm{vd}_{\mathrm{bus},1}$
      | Automatically generated on 2025-11-01 18:39:24 .
  Alge_iq_bus_1_d0ef3 : Inport
  State_vd_bus_1_0a414 : Inport  Port=2
  Constant_15079.644737231_cd7e5 : Constant  Value=15079.644737231
  Constant_376.991118430775_bc05e : Constant  Value=376.991118430775
  Product_97300 : Product
  Product_b4684 : Product
  Subtract_3e947 : Sum  Inputs=+-
  Blockout_d_vq_bus_1_b6261 : Outport
  wires:
  Alge_iq_bus_1_d0ef3/1 -> Product_97300/2
  Constant_15079.644737231_cd7e5/1 -> Product_97300/1
  Product_b4684/1 -> Subtract_3e947/2
  Constant_376.991118430775_bc05e/1 -> Product_b4684/1
  State_vd_bus_1_0a414/1 -> Product_b4684/2
  Product_97300/1 -> Subtract_3e947/1
  Subtract_3e947/1 -> Blockout_d_vq_bus_1_b6261/1

== system IEEE30_case/AC_1/d_vq_bus_20_block ==
  note: d_vq_bus_20 in IEEE30_case
      | $37699111.8430775\,\mathrm{iq}_{\mathrm{bus},20}-376.991118430775\,\mathrm{vd}_{\mathrm{bus},20}$
      | Automatically generated on 2025-11-01 18:39:56 .
  Alge_iq_bus_20_dac44 : Inport
  State_vd_bus_20_3ae12 : Inport  Port=2
  Constant_376.991118430775_f177f : Constant  Value=376.991118430775
  Constant_37699111.8430775_3c39c : Constant  Value=37699111.8430775
  Product_e9e6c : Product
  Product_fcb89 : Product
  Subtract_3c627 : Sum  Inputs=+-
  Blockout_d_vq_bus_20_225c5 : Outport
  wires:
  Constant_37699111.8430775_3c39c/1 -> Product_fcb89/1
  Alge_iq_bus_20_dac44/1 -> Product_fcb89/2
  Product_e9e6c/1 -> Subtract_3c627/2
  Constant_376.991118430775_f177f/1 -> Product_e9e6c/1
  Product_fcb89/1 -> Subtract_3c627/1
  State_vd_bus_20_3ae12/1 -> Product_e9e6c/2
  Subtract_3c627/1 -> Blockout_d_vq_bus_20_225c5/1

== system IEEE30_case/AC_1/d_vq_bus_21_block ==
  note: d_vq_bus_21 in IEEE30_case
      | $37699111.8430775\,\mathrm{iq}_{\mathrm{bus},21}-376.991118430775\,\mathrm{vd}_{\mathrm{bus},21}$
      | Automatically generated on 2025-11-01 18:39:58 .
  Alge_iq_bus_21_81fa7 : Inport
  State_vd_bus_21_a8899 : Inport  Port=2
  Constant_376.991118430775_c6e64 : Constant  Value=376.991118430775
  Constant_37699111.8430775_06e28 : Constant  Value=37699111.8430775
  Product_b98c9 : Product
  Product_bb578 : Product
  Subtract_e39f1 : Sum  Inputs=+-
  Blockout_d_vq_bus_21_3dcf9 : Outport
  wires:
  Constant_37699111.8430775_06e28/1 -> Product_b98c9/1
  Product_bb578/1 -> Subtract_e39f1/2
  Constant_376.991118430775_c6e64/1 -> Product_bb578/1
  Alge_iq_bus_21_81fa7/1 -> Product_b98c9/2
  State_vd_bus_21_a8899/1 -> Product_bb578/2
  Product_b98c9/1 -> Subtract_e39f1/1
  Subtract_e39f1/1 -> Blockout_d_vq_bus_21_3dcf9/1

== system IEEE30_case/AC_1/d_vq_bus_22_block ==
  note: d_vq_bus_22 in IEEE30_case
      | $37699111.8430775\,\mathrm{iq}_{\mathrm{bus},22}-376.991118430775\,\mathrm{vd}_{\mathrm{bus},22}$
      | Automatically generated on 2025-11-01 18:39:59 .
  Alge_iq_bus_22_4e114 : Inport
  State_vd_bus_22_2b8c2 : Inport  Port=2
  Constant_376.991118430775_46f6d : Constant  Value=376.991118430775
  Constant_37699111.8430775_2b1b5 : Constant  Value=37699111.8430775
  Product_37f23 : Product
  Product_c5f93 : Product
  Subtract_66c28 : Sum  Inputs=+-
  Blockout_d_vq_bus_22_04fe2 : Outport
  wires:
  Subtract_66c28/1 -> Blockout_d_vq_bus_22_04fe2/1
  Constant_37699111.8430775_2b1b5/1 -> Product_c5f93/1
  Alge_iq_bus_22_4e114/1 -> Product_c5f93/2
  Constant_376.991118430775_46f6d/1 -> Product_37f23/1
  Product_c5f93/1 -> Subtract_66c28/1
  State_vd_bus_22_2b8c2/1 -> Product_37f23/2
  Product_37f23/1 -> Subtract_66c28/2
